simulink model "EXT_RS232_r2019b_v1"  (Simulink 10.0)
settings: Solver=FixedStepDiscrete  StartTime=0.0  StopTime=inf  FixedStep=0.001  RelTol=1e-3  EnableMultiTasking=on
InitFcn:
  | Simulink.defineIntEnumType('DriverStatus', ...
  |     {'NOT_DEF', 'SYS_OFF', 'ENC_TEST', 'START_CALIB', 'RESET_ENC',...
  |  'END_CALIB', 'READY', 'RUN_IDLE', 'JOINT_FORCE', 'EE_FORCE', 'JOINT_POS',...
  |  'JOINT_VEL', 'EE_POS', 'EE_VEL', 'SYS_ERROR'},...
  |     [0;1;2;3;4;5;6;7;8;9;10;11;12;13;14],...
  |     'Description', 'SYS_STATUS defined in the Finite State Machine', ...
  |     'DefaultValue', 'NOT_DEF',...
  |     'StorageType', 'uint16');
  | 
  | Simulink.defineIntEnumType('DriverFails', ...
  |     {'NO_FAILs', 'CALIB_TIMEOUT', 'COMM_TIMEOUT', 'VEL_HIGH_RUN',...
  |  'VEL_HIGH_CALIB', 'UNKNOWN_CMD_RUNMODE',...
  | 'NOT_DEF1', 'NOT_DEF2', 'NOT_DEF3'}, ...
  |     [0;1;2;3;4;5;6;7;8],...
  |     'Description', 'Set of possible fails', ...
  |     'DefaultValue', 'NO_FAILs', ...
  |     'StorageType', 'uint16');
undefined symbols (not defined in the file): system
libraries: RS232 x2
Description:
  | This is the 3DOF first version of the PERCRO's embedded controller on STM32F4 target
settings Model: Creator=carlo  LastModifiedBy=John_Helsing  ModifiedComment=Simplified 3x3 multiplication M2J J2M  SimulationMode=external
settings Model: ModifiedHistory=|
  | Simplified 3x3 multiplication M2J J2M
  | 
  | Simplified 3x3 multiplication M2J J2M
  | 
  | carlo -- Tue Jan 06 10:41:50 2015 -- Version 1.698
  | Clean up cinematics
  | 
  | carlo -- Mon Jan 05 11:26:31 2015 -- Version 1.696
  | Current Test with new current blockset decoder
  | 
  | Added Reset to ENCODER at startup
  | Added Timer High frequency for current control
  | Added non linearity compensation for current sensing
  | Added new constants in driver description
  | Added new block for current mirror in asynch mode
  | Improved Serioal transport to avoid locks
  | 
  | 
  | carlo -- Mon Dec 29 13:51:31 2014 -- Version 1.613
  | 
  | 
  | carlo -- Mon Dec 29 13:51:31 2014 -- Version 1.613
  | 
  | 
  | carlo -- Tue Dec 16 22:59:42 2014 -- Version 1.607
  | 
  | 
  | carlo -- Tue Dec 16 22:59:42 2014 -- Version 1.607
  | 
  | 
  | carlo -- Tue Dec 16 22:59:42 2014 -- Version 1.607
  | 
  | 
  | carlo -- Tue Dec 16 22:59:42 2014 -- Version 1.607
  | 
  | 
  | carlo -- Tue Dec 16 22:59:42 2014 -- Version 1.607
  | 
  | 
  | carlo -- Tue Dec 16 22:59:42 2014 -- Version 1.607
  | 
  | 
  | carlo -- Tue Dec 16 22:54:29 2014 -- Version 1.606
  | Dev version new scheduler
  | 
  | carlo -- Mon Dec 15 09:01:47 2014 -- Version 1.601
  | Image settings and update block comments
  | 
  | carlo -- Mon Dec 15 09:01:47 2014 -- Version 1.601
  | Image settings and update block comments
  | 
  | carlo -- Mon Dec 15 09:01:47 2014 -- Version 1.601
  | Image settings and update block comments
  | 
  | carlo -- Mon Dec 15 09:01:47 2014 -- Version 1.601
  | Image settings and update block comments
  | 
  | carlo -- Mon Dec 15 09:01:47 2014 -- Version 1.601
  | Image settings and update block comments
  | 
  | carlo -- Sun Dec 14 19:07:54 2014 -- Version 1.600
  | Yanmar Test Model
  | 
  | carlo -- Sun Dec 14 15:14:31 2014 -- Version 1.594
  | Implemented basic COM SFunction
  | Splic com and configuration
  | 
  | carlo -- Sun Dec 14 15:14:31 2014 -- Version 1.594
  | Implemented basic COM SFunction
  | Splic com and configuration
  | 
  | carlo -- Sun Dec 14 15:14:31 2014 -- Version 1.594
  | Implemented basic COM SFunction
  | Splic com and configuration
  | 
  | carlo -- Sun Dec 14 15:14:31 2014 -- Version 1.594
  | Implemented basic COM SFunction
  | Splic com and configuration
  | 
  | carlo -- Sun Dec 14 15:14:31 2014 -- Version 1.594
  | Implemented basic COM SFunction
  | Splic com and configuration
  | 
  | carlo -- Sun Dec 14 15:14:31 2014 -- Version 1.594
  | Implemented basic COM SFunction
  | Splic com and configuration
  | 
  | carlo -- Sat Dec 13 19:47:44 2014 -- Version 1.593
  | New version of Velocity controller
  | 
  | carlo -- Sat Dec 13 10:51:45 2014 -- Version 1.590
  | Forked from 41 to initiate motion test on velocity controller
  | 
  | carlo -- Sat Dec 13 10:51:45 2014 -- Version 1.590
  | Forked from 41 to initiate motion test on velocity controller
  | 
  | carlo -- Sat Dec 13 10:51:45 2014 -- Version 1.590
  | Forked from 41 to initiate motion test on velocity controller
  | 
  | carlo -- Wed Dec 10 14:08:57 2014 -- Version 1.589
  | Low Level Controller setup
  | 
  | carlo -- Wed Dec 10 12:53:39 2014 -- Version 1.588
  | 
  | 
  | carlo -- Tue Dec 09 16:57:00 2014 -- Version 1.587
  | 
  | 
  | carlo -- Mon Dec 08 08:19:23 2014 -- Version 1.586
  | Checked FKD online , delta axis orientation and improved few computational aspects
  | 
  | carlo -- Sun Dec 07 17:29:42 2014 -- Version 1.585
  | Saved with high resolution timer. Checked the versus of motor 2 which was inverted. Checked with new board. Now it works.
  | 
  | carlo -- Thu Dec 04 19:37:13 2014 -- Version 1.556
  | Debug on qm_offset
  | 
  | carlo -- Thu Dec 04 19:37:13 2014 -- Version 1.556
  | Debug on qm_offset
  | 
  | carlo -- Thu Dec 04 19:13:33 2014 -- Version 1.555
  | Implemented Delta motorization variables
  | with MAXON 148877 RE40
  | 
  | carlo -- Thu Dec 04 12:31:38 2014 -- Version 1.554
  | ParamDelta update
  | 
  | carlo -- Thu Dec 04 08:25:30 2014 -- Version 1.553
  | Introduced DELTA motor constant and initialization values in scripting at startup
  | 
  | carlo -- Thu Dec 04 07:23:14 2014 -- Version 1.552
  | Added q_reset in state logic for encoder reset at poweron
  | 
  | carlo -- Mon Dec 01 23:34:58 2014 -- Version 1.547
  | 
  | 
  | carlo -- Mon Dec 01 23:34:58 2014 -- Version 1.547
  | 
  | 
  | carlo -- Mon Dec 01 23:34:58 2014 -- Version 1.547
  | 
  | 
  | carlo -- Mon Dec 01 23:34:58 2014 -- Version 1.547
  | 
  | 
  | carlo -- Mon Dec 01 23:34:58 2014 -- Version 1.547
  | 
  | 
  | carlo -- Mon Dec 01 23:34:15 2014 -- Version 1.546
  | This version implement Delta Kinematics and comments the old GRAB one
  | 
  | Delta cinematics is not yet fully optimized.
  | 
  | 
  | carlo -- Sat Nov 29 11:49:13 2014 -- Version 1.543
  | first documented models with version logging.
  | 
  | carlo -- Sat Nov 29 11:49:13 2014 -- Version 1.543
  | Dirst documented models with version logging.
  | 
  | Release 542:
  |    - Working Encoders
  |    - Working Serial USB transport (base)
  |    - Working Digital OUT
  |    - Working Analog IN
  |    - Working Hbrdges
  |    - Working USB debug
settings DataIOCC: LimitDataPoints=on  SaveOutput=off  SaveTime=off
settings OptimizationCC: DefaultUnderspecifiedDataType=single  ExpressionDepthLimit=2147483647  SimCompilerOptimization=on
settings DebuggingCC: ReadBeforeWriteMsg=DisableAll  WriteAfterWriteMsg=DisableAll  WriteAfterReadMsg=DisableAll  UnderspecifiedInitializationDetection=Simplified  MergeDetectMultiDrivingBlocksExec=error  SolverPrmCheckMsg=warning  InheritedTsInSrcMsg=none  MultiTaskDSMMsg=none  MultiTaskCondExecSysMsg=none  ParameterPrecisionLossMsg=none  FcnCallInpInsideContextMsg=warning  StateNameClashWarn=warning
settings HardwareCC: ProdBitPerPointer=64  ProdBitPerSizeT=64  ProdBitPerPtrDiffT=64  ProdLargestAtomicFloat=Float  ProdIntDivRoundTo=Zero  ProdEndianess=LittleEndian  ProdWordSize=64  ProdHWDeviceType=Intel->x86-64 (Windows64)  TargetBitPerInt=16  TargetBitPerPointer=16  TargetIntDivRoundTo=Zero  TargetEndianess=LittleEndian  TargetWordSize=16  TargetHWDeviceType=STMicroelectronics->ST10/Super10
settings ModelReferenceCC: UpdateModelReferenceTargets=IfOutOfDate
settings SFSimCC: SFSimEcho=off
settings RTWCC: CustomInclude=C:\Users\John_Helsing\Documents\Mechatronics\HAL_STM32F7_March_2017\RS232_For_Matlab-master\Simulink  CustomLibrary=C:\Users\John_Helsing\Documents\Mechatronics\HAL_STM32F7_March_2017\RS232_For_Matlab-master\Simulink\RS232.lib
settings CodeAppCC: MATLABSourceComments=on
settings GRTTargetCC: GeneratePreprocessorConditionals=Disable all  CombineOutputUpdateFcns=on  GRTInterface=off  ExtMode=on
settings ConfigComp: CovExternalEMLEnable=off

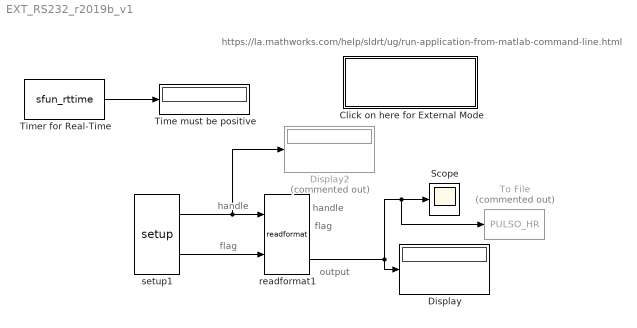
== system EXT_RS232_r2019b_v1 ==
  note: https://la.mathworks.com/help/sldrt/ug/run-application-from-matlab-command-line.html
  note: output
  note: handle
  note: flag
  note: flag
  note: handle
  "Click on here for External Mode " : Subsystem  StartFcn=system(['start ' bdroot '.exe' ])
      settings: OpenFcn=|
      | set_param(gcs,'SimulationMode','external');
      | set_param(gcs,'SimulationCommand','connect');
      mask Display:
      | disp(['Click to connect\n',...
      |   'External Mode\n'...
      | 	  '(double-click)'])
  Display : Display
  Display2 : Display  Commented=on
  Scope : Scope
  Time must be positive : Display
  Timer for Real-Time : S-Function  FunctionName=sfun_rttime  Parameters=1  SFunctionDeploymentMode=off  EnableBusSupport=off
  To File : ToFile  Commented=on  Filename=PULSO_HR  MatrixName=Datos
  readformat1 : RS232/readformat  fmtString=UAEM %d\r\n  nCharTerm=2  sampTime=-1
  setup1 : RS232/setup  port=COM4  baudrate=230400  databit=8  stopbit=1  parity=None
  wires:
  Timer for Real-Time/1 -> Time must be positive/1
  setup1/1 -> readformat1/1, Display2/1
  readformat1/3 -> To File/1, Scope/1, Display/1
  setup1/2 -> readformat1/2

== system EXT_RS232_r2019b_v1/Click on here for External Mode  ==
